simulink model "chan_snap_v3"  (R2012b)
settings: Solver=ode45  StartTime=0.0  StopTime=10000  RelTol=1e-3
undefined symbols (not defined in the file): pfb_coeff_gen_calc, xlipgetpartsetting
libraries: xbsIndex_r4 x7452, casper_library_misc x131, casper_library_flow_control x107, casper_library_delays x40, xps_library x8
(part 2 of 84)

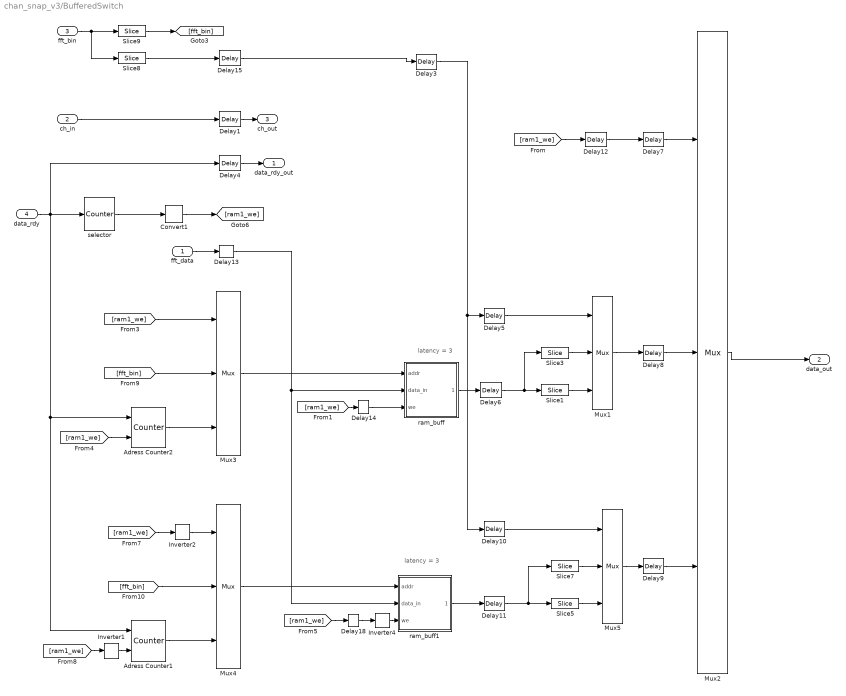
== system chan_snap_v3/BufferedSwitch ==
  note: latency = 3
  note: latency = 3
  fft_data : Inport
  ch_in : Inport  Port=2
  fft_bin : Inport  Port=3
  data_rdy : Inport  Port=4
  Adress Counter1 : xbsIndex_r4/Counter  cnt_type=Free Running  cnt_to=Inf  operation=Up  start_count=0  cnt_by_val=1  arith_type=Unsigned  n_bits=8  bin_pt=0  load_pin=off  rst=on  en=on  explicit_period=on  period=1  dbl_ovrd=off  use_behavioral_HDL=off  implementation=Fabric  use_rpm=off  block_type=counter
  Adress Counter2 : xbsIndex_r4/Counter  cnt_type=Free Running  cnt_to=Inf  operation=Up  start_count=0  cnt_by_val=1  arith_type=Unsigned  n_bits=8  bin_pt=0  load_pin=off  rst=on  en=on  explicit_period=on  period=1  dbl_ovrd=off  use_behavioral_HDL=off  implementation=Fabric  use_rpm=off  block_type=counter
  Convert1 : xbsIndex_r4/Convert  gui_display_data_type=Fixed-point  arith_type=Boolean  n_bits=16  bin_pt=14  float_type=Single  exp_bits=8  fraction_bits=24  quantization=Truncate  overflow=Wrap  en=off  latency=0  dbl_ovrd=off  pipeline=off  block_type=convert
      settings: block_version=10.1.3
  Delay1 : xbsIndex_r4/Delay  rst=off  infoeditControl=Selection of Reset will increase slice count due to use of real FFs and instead of SRLs  en=off  latency=7+256  dbl_ovrd=off  reg_retiming=off  block_type=delay
  Delay{5..6,10..11,13..15,18} (8 alike) : xbsIndex_r4/Delay  rst=off  infoeditControl=Selection of Reset will increase slice count due to use of real FFs and instead of SRLs  en=off  latency=1  dbl_ovrd=off  reg_retiming=off  block_type=delay
  Delay12 : xbsIndex_r4/Delay  rst=off  infoeditControl=Selection of Reset will increase slice count due to use of real FFs and instead of SRLs  en=off  latency=5  dbl_ovrd=off  reg_retiming=off  block_type=delay
  Delay3 : xbsIndex_r4/Delay  rst=off  infoeditControl=Selection of Reset will increase slice count due to use of real FFs and instead of SRLs  en=off  latency=3  dbl_ovrd=off  reg_retiming=off  block_type=delay
  Delay4 : xbsIndex_r4/Delay  rst=off  infoeditControl=Selection of Reset will increase slice count due to use of real FFs and instead of SRLs  en=off  latency=7+256  dbl_ovrd=off  reg_retiming=off  block_type=delay
  Delay7 : xbsIndex_r4/Delay  rst=off  infoeditControl=Selection of Reset will increase slice count due to use of real FFs and instead of SRLs  en=off  latency=2  dbl_ovrd=off  reg_retiming=off  block_type=delay
  Delay8 : xbsIndex_r4/Delay  rst=off  infoeditControl=Selection of Reset will increase slice count due to use of real FFs and instead of SRLs  en=off  latency=2  dbl_ovrd=off  reg_retiming=off  block_type=delay
  Delay9 : xbsIndex_r4/Delay  rst=off  infoeditControl=Selection of Reset will increase slice count due to use of real FFs and instead of SRLs  en=off  latency=2  dbl_ovrd=off  reg_retiming=off  block_type=delay
  Inverter1 : xbsIndex_r4/Inverter  en=off  latency=0  dbl_ovrd=off  block_type=inv
  Inverter2 : xbsIndex_r4/Inverter  en=off  latency=0  dbl_ovrd=off  block_type=inv
  Inverter4 : xbsIndex_r4/Inverter  en=off  latency=0  dbl_ovrd=off  block_type=inv
  Mux1 : xbsIndex_r4/Mux  inputs=2  en=off  latency=0  precision=Full  arith_type=Unsigned  n_bits=16  bin_pt=14  quantization=Truncate  overflow=Wrap  dbl_ovrd=off  block_type=mux
  Mux2 : xbsIndex_r4/Mux  inputs=2  en=off  latency=0  precision=Full  arith_type=Unsigned  n_bits=16  bin_pt=14  quantization=Truncate  overflow=Wrap  dbl_ovrd=off  block_type=mux
  Mux3 : xbsIndex_r4/Mux  inputs=2  en=off  latency=1  precision=Full  arith_type=Unsigned  n_bits=16  bin_pt=14  quantization=Truncate  overflow=Wrap  dbl_ovrd=off  block_type=mux
  Mux4 : xbsIndex_r4/Mux  inputs=2  en=off  latency=1  precision=Full  arith_type=Unsigned  n_bits=16  bin_pt=14  quantization=Truncate  overflow=Wrap  dbl_ovrd=off  block_type=mux
  Mux5 : xbsIndex_r4/Mux  inputs=2  en=off  latency=0  precision=Full  arith_type=Unsigned  n_bits=16  bin_pt=14  quantization=Truncate  overflow=Wrap  dbl_ovrd=off  block_type=mux
  Slice1 : xbsIndex_r4/Slice  nbits=72  boolean_output=off  mode=Lower Bit Location + Width  bit1=0  base1=MSB of Input  bit0=72  base0=LSB of Input  dbl_ovrd=off  block_type=slice
      settings: block_version=10.1.3
  Slice3 : xbsIndex_r4/Slice  nbits=72  boolean_output=off  mode=Lower Bit Location + Width  bit1=0  base1=MSB of Input  bit0=0  base0=LSB of Input  dbl_ovrd=off  block_type=slice
      settings: block_version=10.1.3
  Slice5 : xbsIndex_r4/Slice  nbits=72  boolean_output=off  mode=Lower Bit Location + Width  bit1=0  base1=MSB of Input  bit0=72  base0=LSB of Input  dbl_ovrd=off  block_type=slice
      settings: block_version=10.1.3
  Slice7 : xbsIndex_r4/Slice  nbits=72  boolean_output=off  mode=Lower Bit Location + Width  bit1=0  base1=MSB of Input  bit0=0  base0=LSB of Input  dbl_ovrd=off  block_type=slice
      settings: block_version=10.1.3
  Slice8 : xbsIndex_r4/Slice  nbits=1  boolean_output=off  mode=Lower Bit Location + Width  bit1=0  base1=MSB of Input  bit0=0  base0=LSB of Input  dbl_ovrd=off  block_type=slice
      settings: block_version=10.1.3
  Slice9 : xbsIndex_r4/Slice  nbits=8  boolean_output=off  mode=Lower Bit Location + Width  bit1=0  base1=MSB of Input  bit0=1  base0=LSB of Input  dbl_ovrd=off  block_type=slice
      settings: block_version=10.1.3
  ram_buff : Subsystem
  ram_buff1 : Subsystem
  selector : xbsIndex_r4/Counter  cnt_type=Free Running  cnt_to=Inf  operation=Up  start_count=0  cnt_by_val=1  arith_type=Unsigned  n_bits=1  bin_pt=0  load_pin=off  rst=off  en=on  explicit_period=on  period=1  dbl_ovrd=off  use_behavioral_HDL=off  implementation=Fabric  use_rpm=off  block_type=counter
  data_rdy_out : Outport
  data_out : Outport  Port=2
  ch_out : Outport  Port=3
  wires:
  Mux5/1 -> Delay9/1
  Slice5/1 -> Mux5/3
  Slice7/1 -> Mux5/2
  Slice1/1 -> Mux1/3
  Slice3/1 -> Mux1/2
  Slice9/1 -> [fft_bin]
  Delay4/1 -> data_rdy_out/1
  fft_bin/1 -> Slice9/1, Slice8/1
  Slice8/1 -> Delay15/1
  Delay3/1 -> Delay5/1, Delay10/1
  Mux1/1 -> Delay8/1
  Convert1/1 -> [ram1_we]
  Mux2/1 -> data_out/1
  Delay9/1 -> Mux2/3
  Delay8/1 -> Mux2/2
  Delay7/1 -> Mux2/1
  [ram1_we] -> Delay18/1
  Inverter2/1 -> Mux4/1
  [ram1_we] -> Inverter2/1
  Inverter1/1 -> Adress Counter1/2
  [ram1_we] -> Inverter1/1
  [fft_bin] -> Mux4/2
  Adress Counter1/1 -> Mux4/3
  data_rdy/1 -> selector/1, Adress Counter1/1, Adress Counter2/1, Delay4/1
  [fft_bin] -> Mux3/2
  Adress Counter2/1 -> Mux3/3
  [ram1_we] -> Mux3/1
  [ram1_we] -> Delay12/1
  [ram1_we] -> Adress Counter2/2
  selector/1 -> Convert1/1
  Delay1/1 -> ch_out/1
  ch_in/1 -> Delay1/1
  Delay5/1 -> Mux1/1
  Delay10/1 -> Mux5/1
  Delay6/1 -> Slice1/1, Slice3/1
  Delay11/1 -> Slice7/1, Slice5/1
  Delay12/1 -> Delay7/1
  fft_data/1 -> Delay13/1
  Delay15/1 -> Delay3/1
  ram_buff/1(data_out) -> Delay6/1
  ram_buff1/1(data_out) -> Delay11/1
  Delay13/1 -> ram_buff1/2(data_in), ram_buff/2(data_in)
  Mux3/1 -> ram_buff/1(addr)
  [ram1_we] -> Delay14/1
  Inverter4/1 -> ram_buff1/3(we)
  Mux4/1 -> ram_buff1/1(addr)
  Delay14/1 -> ram_buff/3(we)
  Delay18/1 -> Inverter4/1

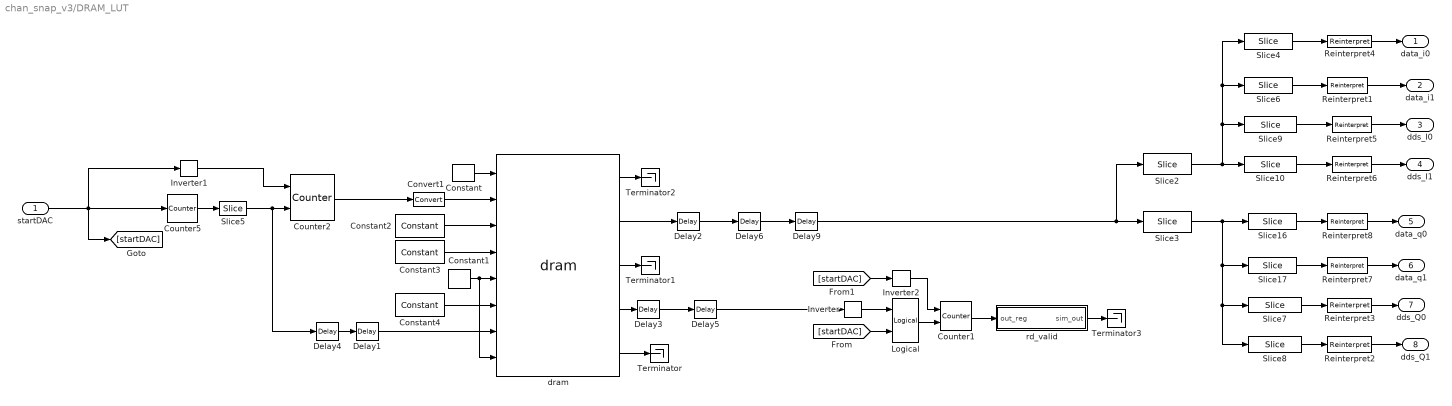
== system chan_snap_v3/DRAM_LUT ==
  startDAC : Inport
  Constant : xbsIndex_r4/Constant  const=0  gui_display_data_type=Fixed-point  arith_type=Boolean  n_bits=16  bin_pt=14  preci_type=Single  exp_width=8  frac_width=24  explicit_period=on  period=1  equ=P=C  opselect=C  inp2=PCIN>>17  opr=+  inp1=P  carry=CIN  dbl_ovrd=off  block_type=constant
  Constant1 : xbsIndex_r4/Constant  const=1  gui_display_data_type=Fixed-point  arith_type=Boolean  n_bits=16  bin_pt=14  preci_type=Single  exp_width=8  frac_width=24  explicit_period=on  period=1  equ=P=C  opselect=C  inp2=PCIN>>17  opr=+  inp1=P  carry=CIN  dbl_ovrd=off  block_type=constant
  Constant2 : xbsIndex_r4/Constant  const=0  gui_display_data_type=Fixed-point  arith_type=Unsigned  n_bits=144  bin_pt=0  preci_type=Single  exp_width=8  frac_width=24  explicit_period=on  period=1  equ=P=C  opselect=C  inp2=PCIN>>17  opr=+  inp1=P  carry=CIN  dbl_ovrd=off  block_type=constant
  Constant3 : xbsIndex_r4/Constant  const=0  gui_display_data_type=Fixed-point  arith_type=Unsigned  n_bits=36  bin_pt=0  preci_type=Single  exp_width=8  frac_width=24  explicit_period=on  period=1  equ=P=C  opselect=C  inp2=PCIN>>17  opr=+  inp1=P  carry=CIN  dbl_ovrd=off  block_type=constant
  Constant4 : xbsIndex_r4/Constant  const=0  gui_display_data_type=Fixed-point  arith_type=Unsigned  n_bits=32  bin_pt=0  preci_type=Single  exp_width=8  frac_width=24  explicit_period=on  period=1  equ=P=C  opselect=C  inp2=PCIN>>17  opr=+  inp1=P  carry=CIN  dbl_ovrd=off  block_type=constant
  Convert1 : xbsIndex_r4/Convert  gui_display_data_type=Fixed-point  arith_type=Unsigned  n_bits=32  bin_pt=0  float_type=Single  exp_bits=8  fraction_bits=24  quantization=Truncate  overflow=Wrap  en=off  latency=0  dbl_ovrd=off  pipeline=off  block_type=convert
      settings: block_version=11.4
  Counter1 : xbsIndex_r4/Counter  cnt_type=Free Running  cnt_to=511  operation=Up  start_count=0  cnt_by_val=1  arith_type=Unsigned  n_bits=14  bin_pt=0  load_pin=off  rst=on  en=on  explicit_period=on  period=1  dbl_ovrd=off  use_behavioral_HDL=off  implementation=Fabric  use_rpm=off  block_type=counter
  Counter2 : xbsIndex_r4/Counter  cnt_type=Free Running  cnt_to=512  operation=Up  start_count=0  cnt_by_val=1  arith_type=Unsigned  n_bits=14  bin_pt=0  load_pin=off  rst=on  en=on  explicit_period=on  period=1  dbl_ovrd=off  use_behavioral_HDL=off  implementation=Fabric  use_rpm=off  block_type=counter
  Counter5 : xbsIndex_r4/Counter  cnt_type=Free Running  cnt_to=511  operation=Up  start_count=0  cnt_by_val=1  arith_type=Unsigned  n_bits=1  bin_pt=0  load_pin=off  rst=off  en=on  explicit_period=on  period=1  dbl_ovrd=off  use_behavioral_HDL=off  implementation=Fabric  use_rpm=off  block_type=counter
  Delay{1..4} (4 alike) : xbsIndex_r4/Delay  rst=off  infoeditControl=Selection of Reset will increase slice count due to use of real FFs and instead of SRLs  en=off  latency=2  dbl_ovrd=off  reg_retiming=off  block_type=delay
  Delay5 : xbsIndex_r4/Delay  rst=off  infoeditControl=Selection of Reset will increase slice count due to use of real FFs and instead of SRLs  en=off  latency=1  dbl_ovrd=off  reg_retiming=off  block_type=delay
  Delay6 : xbsIndex_r4/Delay  rst=off  infoeditControl=Selection of Reset will increase slice count due to use of real FFs and instead of SRLs  en=off  latency=1  dbl_ovrd=off  reg_retiming=off  block_type=delay
  Delay9 : xbsIndex_r4/Delay  rst=off  infoeditControl=Selection of Reset will increase slice count due to use of real FFs and instead of SRLs  en=off  latency=1  dbl_ovrd=off  reg_retiming=off  block_type=delay
  Inverter : xbsIndex_r4/Inverter  en=off  latency=0  dbl_ovrd=off  block_type=inv
      settings: block_version=11.4
  Inverter1 : xbsIndex_r4/Inverter  en=off  latency=0  dbl_ovrd=off  block_type=inv
      settings: block_version=11.4
  Inverter2 : xbsIndex_r4/Inverter  en=off  latency=0  dbl_ovrd=off  block_type=inv
      settings: block_version=11.4
  Logical : xbsIndex_r4/Logical  logical_function=AND  inputs=2  en=off  latency=0  precision=Full  arith_type=Unsigned  n_bits=16  bin_pt=0  align_bp=on  dbl_ovrd=off  block_type=logical
      settings: block_version=11.4
  Reinterpret{1..8} (8 alike) : xbsIndex_r4/Reinterpret  force_arith_type=on  arith_type="Signed  (2's comp)"  force_bin_pt=on  bin_pt=15  block_type=reinterpret
      settings: infoedit="Changes signal type without altering the binary representation.   You can changed the signal between signed and unsigned, and relocate the binary point.<P><P>Hardware notes: In hardware this block costs nothing.<P><P>Example:  Suppose the input is 6 bits wide, signed, with 2 fractional bits, and the output is forced to unsigned with 0 fractional bits.  Then an input of -2.0 (1110.00 in binary 2's complement) becomes an output of 56 (111000 in binary)."  block_version=10.1.3
  Slice10 : xbsIndex_r4/Slice  nbits=16  boolean_output=off  mode=Lower Bit Location + Width  bit1=0  base1=MSB of Input  bit0=48  base0=LSB of Input  dbl_ovrd=off  block_type=slice
      settings: block_version=10.1.3
  Slice16 : xbsIndex_r4/Slice  nbits=16  boolean_output=off  mode=Lower Bit Location + Width  bit1=0  base1=MSB of Input  bit0=0  base0=LSB of Input  dbl_ovrd=off  block_type=slice
      settings: block_version=10.1.3
  Slice17 : xbsIndex_r4/Slice  nbits=16  boolean_output=off  mode=Lower Bit Location + Width  bit1=0  base1=LSB of Input  bit0=16  base0=LSB of Input  dbl_ovrd=off  block_type=slice
      settings: block_version=10.1.3
  Slice2 : xbsIndex_r4/Slice  nbits=64  boolean_output=off  mode=Lower Bit Location + Width  bit1=0  base1=MSB of Input  bit0=0  base0=LSB of Input  dbl_ovrd=off  block_type=slice
      settings: block_version=10.1.3
  Slice3 : xbsIndex_r4/Slice  nbits=64  boolean_output=off  mode=Lower Bit Location + Width  bit1=0  base1=MSB of Input  bit0=72  base0=LSB of Input  dbl_ovrd=off  block_type=slice
      settings: block_version=10.1.3
  Slice4 : xbsIndex_r4/Slice  nbits=16  boolean_output=off  mode=Lower Bit Location + Width  bit1=0  base1=MSB of Input  bit0=0  base0=LSB of Input  dbl_ovrd=off  block_type=slice
      settings: block_version=10.1.3
  Slice5 : xbsIndex_r4/Slice  nbits=1  boolean_output=on  mode=Lower Bit Location + Width  bit1=0  base1=MSB of Input  bit0=0  base0=LSB of Input  dbl_ovrd=off  block_type=slice
      settings: block_version=10.1.3
  Slice6 : xbsIndex_r4/Slice  nbits=16  boolean_output=off  mode=Lower Bit Location + Width  bit1=0  base1=LSB of Input  bit0=16  base0=LSB of Input  dbl_ovrd=off  block_type=slice
      settings: block_version=10.1.3
  Slice7 : xbsIndex_r4/Slice  nbits=16  boolean_output=off  mode=Lower Bit Location + Width  bit1=0  base1=MSB of Input  bit0=32  base0=LSB of Input  dbl_ovrd=off  block_type=slice
      settings: block_version=10.1.3
  Slice8 : xbsIndex_r4/Slice  nbits=16  boolean_output=off  mode=Lower Bit Location + Width  bit1=0  base1=MSB of Input  bit0=48  base0=LSB of Input  dbl_ovrd=off  block_type=slice
      settings: block_version=10.1.3
  Slice9 : xbsIndex_r4/Slice  nbits=16  boolean_output=off  mode=Lower Bit Location + Width  bit1=0  base1=MSB of Input  bit0=32  base0=LSB of Input  dbl_ovrd=off  block_type=slice
      settings: block_version=10.1.3
  Terminator{,1..3} (4 alike) : Terminator
  dram : xps_library/dram  Tag=xps:dram  dimm=1  arith_type=Unsigned  bin_pt=0  ip_clock=266  sample_period=1  bram_fifos=on  disable_tag=off  ram_depth=18  bank_mgt=off  wide_data=off  half_burst=off  use_sniffer=on
      link override convert_data_in: arith_type=Unsigned  n_bits=144  bin_pt=0
      link override convert_wr_be: n_bits=18
      link override ddc256_4x_nofir_snap_DRAM_LUT_dram_Mem_Rd_Dout: n_bits=144
      link override ddc256_4x_snap2_DRAM_LUT_dram_Mem_Rd_Dout: n_bits=144
      link override ddc256_4x_snap_fir_DRAM_LUT_dram_Mem_Rd_Dout: n_bits=144
      link override force_rd_dout: arith_type=Unsigned  bin_pt=0
      link override sim_wrapper/dram_sim: sim_method=Inactive  engine_block=ModelSim
  rd_valid : Subsystem  Tag=xps:sw_reg  AncestorBlock=xps_library/software register  mask{numios=1, io_dir=To Processor, io_delay=0, sample_period=1, name1=reg, bitwidth1=32, arith_type1=Unsigned, bin_pt1=0}
      mask prompts: numios "Num I/Os"; io_dir "I/O direction"; io_delay "I/O delay"; sample_period "Sample period"; name1 "Name"; bitwidth1 "Bitwidth"; arith_type1 "Type"; bin_pt1 "Binary pt"
      mask init:
      | swreg_init(gcb);
      mask Callback numios: t = timer('StartDelay', 0.1); t.TimerFcn = {@swreg_cb, gcb}; start(t);
      mask TypeOptions io_dir: To Processor | From Processor
      mask Callback io_dir:
      | a = get_param(gcb, 'MaskEnables');
      | if strcmp(get_param(gcb, 'io_dir'), 'To Processor'),
      | a(4) = {'off'};
      | else
      | a(4) = {'on'};
      | end
      | set_param(gcb, 'MaskEnables', a);
      mask TypeOptions arith_type1: Unsigned | Signed  (2's comp) | Boolean
      mask Callback arith_type1:
      | a = get_param(gcb, 'MaskEnables');
      | if strcmp(get_param(gcb, 'arith_type1'), 'Boolean'),
      | set_param(gcb, 'bitwidth1', '1');
      | set_param(gcb, 'bin_pt1', '0');
      | a(6) = {'off'};
      | a(8) = {'off'};
      | else
      | a(6) = {'on'};
      | a(8) = {'on'};
      | end
      | set_param(gcb, 'MaskEnables', a);
  data_i0 : Outport
  data_i1 : Outport  Port=2
  dds_I0 : Outport  Port=3
  dds_I1 : Outport  Port=4
  data_q0 : Outport  Port=5
  data_q1 : Outport  Port=6
  dds_Q0 : Outport  Port=7
  dds_Q1 : Outport  Port=8
  wires:
  Constant/1 -> dram/1
  Constant1/1 -> dram/8, dram/5
  Constant2/1 -> dram/3
  Constant3/1 -> dram/4
  Slice5/1 -> Counter2/2, Delay4/1
  dram/4 -> Delay3/1
  Constant4/1 -> dram/6
  Delay4/1 -> Delay1/1
  Slice4/1 -> Reinterpret4/1
  Slice6/1 -> Reinterpret1/1
  Slice9/1 -> Reinterpret5/1
  Slice10/1 -> Reinterpret6/1
  Reinterpret4/1 -> data_i0/1
  Reinterpret1/1 -> data_i1/1
  Reinterpret5/1 -> dds_I0/1
  Reinterpret6/1 -> dds_I1/1
  Reinterpret8/1 -> data_q0/1
  Reinterpret7/1 -> data_q1/1
  Reinterpret3/1 -> dds_Q0/1
  Reinterpret2/1 -> dds_Q1/1
  startDAC/1 -> Counter5/1, [startDAC], Inverter1/1
  Counter5/1 -> Slice5/1
  Inverter/1 -> Logical/1
  [startDAC] -> Logical/2
  Convert1/1 -> dram/2
  Slice16/1 -> Reinterpret8/1
  Slice17/1 -> Reinterpret7/1
  Slice7/1 -> Reinterpret3/1
  Slice8/1 -> Reinterpret2/1
  Slice2/1 -> Slice10/1, Slice9/1, Slice6/1, Slice4/1
  Slice3/1 -> Slice16/1, Slice17/1, Slice7/1, Slice8/1
  Counter1/1 -> rd_valid/1(out_reg)
  Logical/1 -> Counter1/2
  [startDAC] -> Inverter2/1
  Inverter2/1 -> Counter1/1
  dram/2 -> Delay2/1
  Counter2/1 -> Convert1/1
  Inverter1/1 -> Counter2/1
  dram/5 -> Terminator/1
  dram/3 -> Terminator1/1
  dram/1 -> Terminator2/1
  rd_valid/1(sim_out) -> Terminator3/1
  Delay1/1 -> dram/7
  Delay2/1 -> Delay6/1
  Delay9/1 -> Slice3/1, Slice2/1
  Delay3/1 -> Delay5/1
  Delay6/1 -> Delay9/1
  Delay5/1 -> Inverter/1
